simulink model "Parabolas"  (R2018a)
settings: Solver=FixedStepAuto  StartTime=0.0  StopTime=2  FixedStep=0.2  RelTol=1e-3
InitFcn:
  | x = -0.0845;
  | y = 0.1249;
  | altura = 1;
  | Vx = 0;
  | Vy = 0;
  | ace = 0;
  | estado = 0;
libraries: simulink x2
settings Model: Creator=Carlos  LastModifiedBy=Carlos

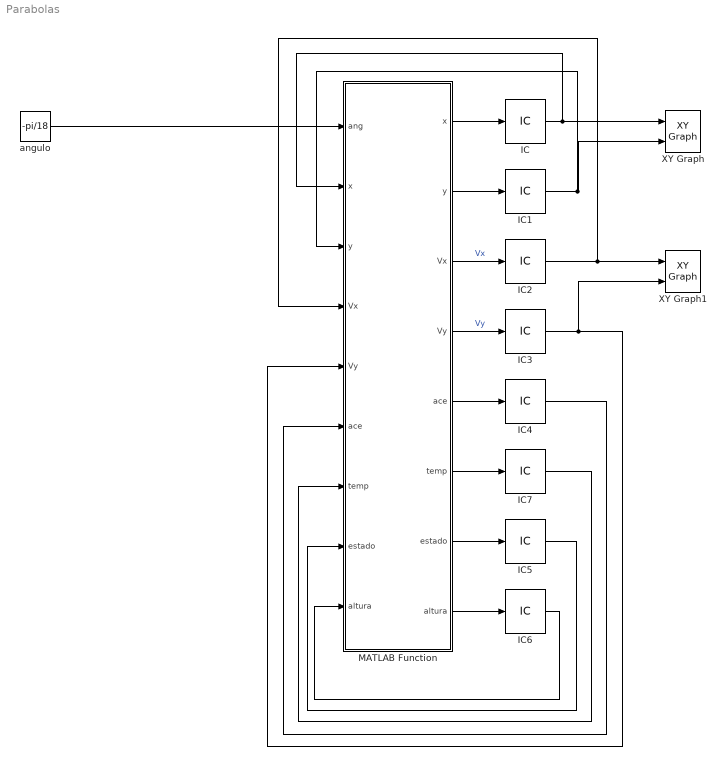
== system Parabolas ==
  IC : InitialCondition  Value=-0.08475
  IC1 : InitialCondition  Value=0.1249
  IC{2..5,7} (5 alike) : InitialCondition  Value=0
  IC6 : InitialCondition
  MATLAB Function : MATLAB Function  TreatAsAtomicUnit=on
  XY Graph : simulink/Sinks/XY Graph  xmin=-1  xmax=1  ymin=-1  ymax=1  st=-1
  XY Graph1 : simulink/Sinks/XY Graph  xmin=-1  xmax=1  ymin=-1  ymax=1  st=-1
  angulo : Constant  Value=-pi/18
  wires:
  IC/1 -> MATLAB Function/2("x "), XY Graph/1
  MATLAB Function/1(x) -> IC/1
  MATLAB Function/2(y) -> IC1/1
  IC1/1 -> MATLAB Function/3("y "), XY Graph/2
  MATLAB Function/3(Vx) -> IC2/1  "Vx"
  IC2/1 -> MATLAB Function/4("Vx "), XY Graph1/1
  MATLAB Function/4(Vy) -> IC3/1  "Vy"
  IC3/1 -> MATLAB Function/5("Vy "), XY Graph1/2
  MATLAB Function/5(ace) -> IC4/1
  MATLAB Function/7(estado) -> IC5/1
  MATLAB Function/8(altura) -> IC6/1
  IC6/1 -> MATLAB Function/9("altura ")
  IC5/1 -> MATLAB Function/8("estado ")
  IC4/1 -> MATLAB Function/6("ace ")
  angulo/1 -> MATLAB Function/1(ang)
  MATLAB Function/6(temp) -> IC7/1
  IC7/1 -> MATLAB Function/7("temp ")

== matlab function Parabolas/MATLAB Function ==
  data: ang input; x output; y output; Vx output; Vy output; x input; y input; Vx input; Vy input; ace input; ace output; temp output; temp input; estado input; estado output; altura input; altura output
function [x,y,Vx,Vy,ace,temp,estado,altura] = Modelo(ang,x,y,Vx,Vy,ace,temp,estado,altura)

    
    %% Definición de variables

    ang
    x
    y
    Vx
    Vy
    ace
    temp = temp + 0.001
    estado
    altura
    
    % Angulo de giro
    ang = -ang;

    % Dificultad
    dif = 4;

    % Altura del carril
    ini = 0.16;
    inc = 0.0457;
    alturas = zeros(1,8);
    for j = 1:4
        alturas(j) = ini - (j-1)*inc;
    end
    for j = 5:8
        alturas(j) = -alturas(9-j);
    end
    alt = alturas(int8(altura)+1);
    
    % Trigonometría
    c = cos(ang);
    s = sin(ang);
    t = tan(ang);
    t = 1/t;
    
    % Vectores de la posición de caida para distintas dificultades
    caida = zeros(4,7,2);
    caida(1,:,:) = [0 0.11429;
               0 0.06857;
               0 0.02286;
               0 -0.02286;
               0 -0.06857;
               0 -0.11429;
               -0.02554 -0.16035];

    caida(2,:,:) = [0.06211 0.11223;
               -0.04758 0.06799;
               0.04969 0.02154;
               -0.04847 -0.02411;
               0.04406 -0.06961;
               -0.05409 -0.11585;
               -0.02554 -0.16035];

    caida(3,:,:) = [0.12394 0.10605;
               -0.09503 0.06374;
               0.09924 0.01759;
               -0.0968 -0.02787;
               0.08803 -0.07271;
               -0.108 -0.12053;
               -0.02554 -0.16035];

    caida(4,:,:) = [0.12394 0.10605;
               -0.14224 0.05771;
               0.14851 0.01102;
               -0.14488 -0.03412;
               0.1318 -0.07789;
               -0.108 -0.12053;
               -0.02554 -0.16035];
           
    %% Lógica del modelo
    if ang~=0
        % Cambio a sistema de referencia no variable
        for j = 1:size(caida,1)
            for k = 1:size(caida,2)
                x = caida(j,k,1);
                y = caida(j,k,2);
                dist = sqrt(x^2+y^2);
                if y>=0
                    gamma = atan(x/y);
                elseif x>=0
                    gamma = pi + atan(x/y);
                else
                    gamma = -pi + atan(x/y);
                end

                caida(j,k,1) = dist*sin(gamma+ang);
                caida(j,k,2) = dist*cos(gamma+ang);
            end
        end

        
        % Valores representativos de la parábola

        % Reducción de complejidad
        a = t - 1/(s*c);
        b = (alt + 0.463)/c;

        % Punto focal
        xF = (alt-0.463)*s;
        yF = (alt-0.463)*c;

        A = 1;
        B = 2*a;
        C = a^2;
        D = -2*(xF*(a^2+1)+b*a);
        E = 2*(b-(a^2+1)*yF);
        F = (a^2+1)*xF^2 + (a^2+1)*yF^2 - b^2;

        % Calculo de la posición en y
        y = (-(B*x+E)+sqrt((B*x+E)^2-4*C*(A*x^2+D*x+F)))/(2*C);
        if (abs(y)>0.25)
            y = (-(B*x+E)-sqrt((B*x+E)^2-4*C*(A*x^2+D*x+F)))/(2*C);
        end

        % Derivada e inclinación de un punto de la parábola
        der = -(2*A*x+B*y+D)/(B*x+2*C*y+E);
        alpha = atan(der);

        % Parámetros del modelo
        g = 9.8;
        R = 0.2325/2;
        m = 7.5e-3;

        % Estudio de la posición, velocidad y aceleración
        V = sqrt(Vx^2+Vy^2);
        pose = mod(altura,2);
        x_1 = x;

        if abs(x)<0.25

            % Caida de la moneda desde un carril al inmediatamente inferior
            if ((((x>=caida(dif,int8(altura),1))&&(caida(dif,int8(altura),1)>0))||((x<=caida(dif,int8(altura),1))&&(caida(dif,int8(altura),1)<0)))||(estado==1))

                if estado == 0
                    estado = 1;
                    altura = altura + 1;
                    alt = alturas(altura+1);
                end
                
                % Calculo del punto de recepción
                valor_func = 1;
                
                x = x + Vx*temp;
                y = y + Vy*temp - 0.5*g*temp^2;
                valor_func = A*x^2+B*x*y+C*y^2+D*x+E*y+F;

                Vy = Vy - g*temp;
                ace = 2*g*sin(-alpha)/3;
                
                if (valor_func<0)
                    
                    estado = 0;
                    
                    % Derivada e inclinación del nuevo punto de la parábola
                    der = -(2*A*x+B*y+D)/(B*x+2*C*y+E);
                    alpha = atan(der);

                    % Velocidades en el punto de recepción
                    Vy = Vx*tan(alpha);
                    V = Vx*sqrt(1+(tan(alpha))^2);
                    
                end

                

            end

            % La caida al siguiente nivel se encuentra a la derecha
            if pose==1

                if x<caida(dif,int8(altura),1)

                    % Nueva posición en x
                    x = x + Vx*temp + 0.5*ace*cos(alpha)*temp^2;
                    
                    % Si se pasa del punto límete se interpola
                    if x>caida(dif,int8(altura),1)
                        gan = (caida(dif,altura,1)-x_1)/(x-x_1);
                        x = caida(dif,altura,1);
                    else
                        gan = 1;
                    end
                    
                    % Calculo de y
                    y = (-(B*x+E)+sqrt((B*x+E)^2-4*C*(A*x^2+D*x+F)))/(2*C);
                    if (abs(y)>0.25)
                        y = (-(B*x+E)-sqrt((B*x+E)^2-4*C*(A*x^2+D*x+F)))/(2*C);
                    end

                    % Inclinación de la nueva posición
                    der = -(2*A*x+B*y+D)/(B*x+2*C*y+E);
                    alpha = atan(der);

                    % Nueva velocidad y sus componentes
                    V = V + gan*ace*temp;
                    Vx = V*cos(alpha);
                    Vy = V*sin(alpha);

                    % Nueva aceleración
                    ace = 2*g*sin(-alpha)/3;

                end

            % La caida al siguiente nivel se encuentra a la derecha
            else

                while x>caida(dif,int8(altura),1)

                    % Nueva posición
                    x = x + Vx*temp + 0.5*ace*cos(alpha)*temp^2;
                    
                    % Si se pasa del punto límete se interpola
                    if x<caida(dif,int8(altura),1)
                        gan = (x_1-caida(dif,altura,1))/(x_1-x);
                        x = caida(dif,altura,1);
                    else
                        gan = 1;
                    end
                    
                    % Calculo de y
                    y = (-(B*x+E)+sqrt((B*x+E)^2-4*C*(A*x^2+D*x+F)))/(2*C);
                    if (abs(y)>0.25)
                        y = (-(B*x+E)-sqrt((B*x+E)^2-4*C*(A*x^2+D*x+F)))/(2*C);
                    end

                    % Inclinación de la nueva posición
                    der = -(2*A*x+B*y+D)/(B*x+2*C*y+E);
                    alpha = atan(der);

                    % Nueva velocidad 
                    V = V + gan*ace*temp;
                    Vx = V*cos(alpha);
                    Vy = V*sin(alpha);

                    % Nueva aceleración
                    ace = 2*g*sin(-alpha)/3;

                end
            end
        end

    else

        a = 0;

    end
